simulink model "rp_modelling_nl"  (R2023b)
settings: Solver=VariableStepAuto  StartTime=0.0  StopTime=rp_p.simtime  RelTol=1e-6  AbsTol=1e-6
values from neighbouring files (symbols this model uses):
  rp_p = rp_parameters()    [rp_mainfile_modelling_comparison_a.m]    (also in rp_mainfile_ofc_comparison_b.m)
undefined symbols (not defined in the file or in its folder): rp_nl_model
settings Model: Creator=gory  LastModifiedBy=cgorman

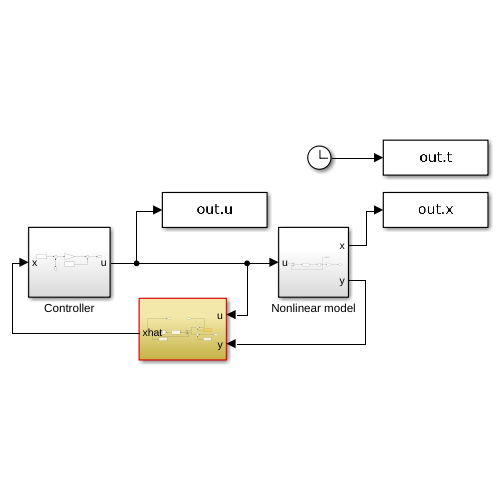
[thumbnail: Simulink's stored preview of the top-level diagram]
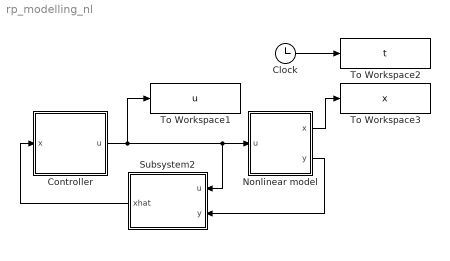
== system rp_modelling_nl ==
  Clock : Clock
  Controller : Subsystem
  Nonlinear model : Subsystem
  Subsystem2 : Subsystem
  To Workspace1 : ToWorkspace  VariableName=u
  To Workspace2 : ToWorkspace  VariableName=t  SampleTime=-1
  To Workspace3 : ToWorkspace  VariableName=x
  wires:
  Clock/1 -> To Workspace2/1
  Nonlinear model/1(x) -> To Workspace3/1
  Controller/1(u) -> Nonlinear model/1(u), Subsystem2/1(u), To Workspace1/1
  Nonlinear model/2(y) -> Subsystem2/2(y)
  Subsystem2/1(xhat) -> Controller/1(x)

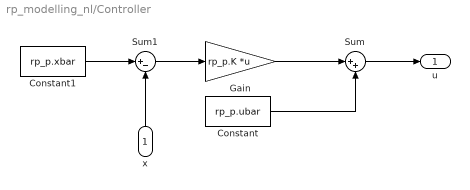
== system rp_modelling_nl/Controller ==
  x : Inport
  Constant : Constant  Value=rp_p.ubar
  Constant1 : Constant  Value=rp_p.xbar
  Gain : Gain  Gain=rp_p.K  Multiplication=Matrix(K*u)
  Sum : Sum  Inputs=|++
  Sum1 : Sum  Inputs=|+-
  u : Outport
  wires:
  Constant/1 -> Sum/2
  Gain/1 -> Sum/1
  Constant1/1 -> Sum1/1
  x/1 -> Sum1/2
  Sum1/1 -> Gain/1
  Sum/1 -> u/1

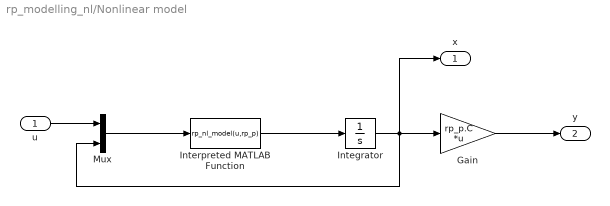
== system rp_modelling_nl/Nonlinear model ==
  u : Inport
  Gain : Gain  Gain=rp_p.C  Multiplication=Matrix(K*u)
  Integrator : Integrator  InitialCondition=rp_p.ic
  Interpreted MATLAB Function : MATLABFcn  MATLABFcn=rp_nl_model(u,rp_p)
  Mux : Mux  Inputs=2
  x : Outport
  y : Outport  Port=2
  wires:
  Interpreted MATLAB Function/1 -> Integrator/1
  Mux/1 -> Interpreted MATLAB Function/1
  Integrator/1 -> x/1, Gain/1, Mux/2
  Gain/1 -> y/1
  u/1 -> Mux/1

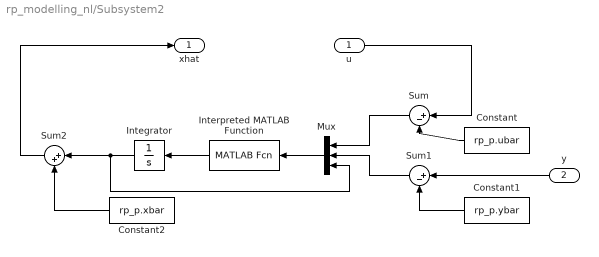
== system rp_modelling_nl/Subsystem2 ==
  u : Inport
  y : Inport  Port=2
  Constant : Constant  Value=rp_p.ubar
  Constant1 : Constant  Value=rp_p.ybar
  Constant2 : Constant  Value=rp_p.xbar
  Integrator : Integrator
  Interpreted MATLAB Function : MATLABFcn
  Mux : Mux  Inputs=3
  Sum : Sum  Inputs=|+-
  Sum1 : Sum  Inputs=|+-
  Sum2 : Sum  Inputs=|++
  xhat : Outport
  wires:
  Mux/1 -> Interpreted MATLAB Function/1
  Sum1/1 -> Mux/2
  Constant2/1 -> Sum2/2
  Sum2/1 -> xhat/1
  Sum/1 -> Mux/1
  Constant/1 -> Sum/2
  Integrator/1 -> Sum2/1, Mux/3
  y/1 -> Sum1/1
  Interpreted MATLAB Function/1 -> Integrator/1
  Constant1/1 -> Sum1/2
  u/1 -> Sum/1
